simulink model "ThdynTest"  (R2013a)
settings: Solver=ode45  StartTime=0  StopTime=1  FixedStep=1e-3  RelTol=1e-5  AbsTol=1e-5
values from neighbouring files (symbols this model uses):
  B = [B1;B2]    [GensetRespOptimiztion.m]    (also in GensetRespOptimiztionTorstein.m; Init8RTFLEX68D.m = 0.68; init_MVM.m = 0.127)
  FExh0 = 0    [Init8RTFLEX68D.m]
  fs = 0.0683    [Init8RTFLEX68D.m]    (also in NOxProcessGUI.m = varargin{2}; initHybrid.m; initMV.m; init_MVM.m = 0.0682925799315)
  FScav0 = 0    [Init8RTFLEX68D.m]
  mCV = p*VCV / (R*T)    [ThdynCVTestScript.m]    (also in ThdynTest.m)
  mfCV = F*fs / (1+F*fs) * mCV    [ThdynCVTestScript.m]    (also in ThdynTest.m)
  pExh0 = pExhRef(caseInit)    [Init8RTFLEX68D.m]
  pScav0 = pScavRef(caseInit)    [Init8RTFLEX68D.m]
  RPM0 = simin(1,2)    [Init8RTFLEX68D.m]
  stroke = 2.72    [Init8RTFLEX68D.m]
  TExh0 = TExhRef(caseInit)    [Init8RTFLEX68D.m]
  TScav0 = TScavRef(caseInit)    [Init8RTFLEX68D.m]
  UCV = u*mCV    [ThdynCVTestScript.m]    (also in ThdynTest.m)
  VCV = 1.2    [ThdynCVTestScript.m]    (also in ThdynTest.m = 1)
undefined symbols (not defined in the file): alpha, beta, cAlpha, cAStartRef, cAVVDownRef, cAVVUpRef, cCylHT, dCALiftDown, dCALiftTopRef, dCALiftUp, Dp, DPhiMix, Ds, Dv, ECyl0, FCyl0, hn, lambdaCrank, liftDownRef, liftMax, liftUpRef, mbCyl0, mCp, mCyl0, mqfCycMax, nCyl, nPort, nStroke, pCyl0, phi0, phi0Mix, r, TCyl0, vCyl0, w, wiebePara, X, Y
libraries: EngineSysteSubmodel x12
settings Model: Creator=yum  LastModifiedBy=yum
settings DataIOCC: SaveFormat=StructureWithTime  ReturnWorkspaceOutputs=on

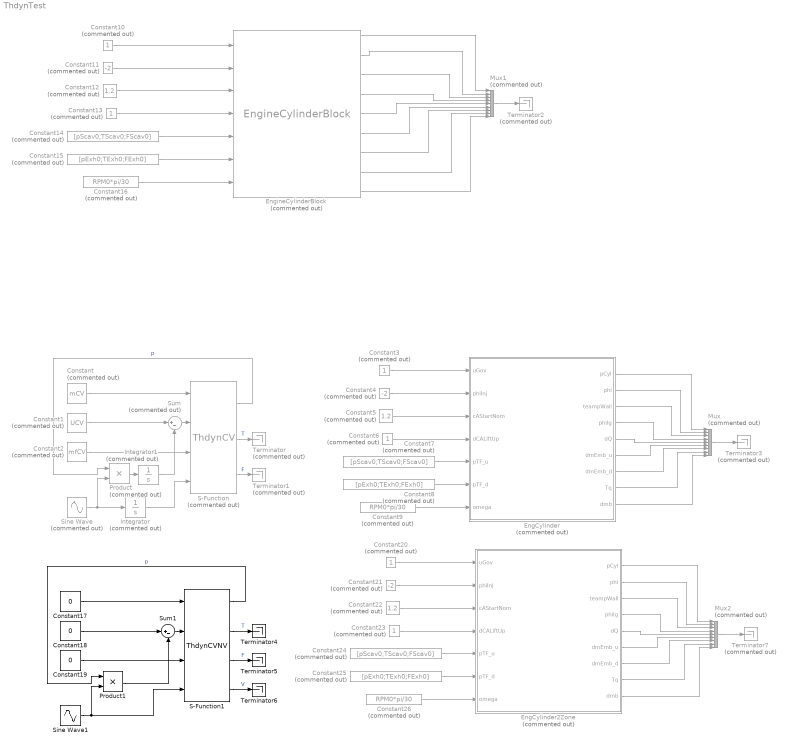
== system ThdynTest ==
  Constant : Constant  Commented=on  Value=mCV
  Constant1 : Constant  Commented=on  Value=UCV
  Constant{3,6,10,13,20,23} (6 alike) : Constant  Commented=on
  Constant11 : Constant  Commented=on  Value=-2
  Constant12 : Constant  Commented=on  Value=1.2
  Constant14 : Constant  Commented=on  Value=[pScav0;TScav0;FScav0]
  Constant15 : Constant  Commented=on  Value=[pExh0;TExh0;FExh0]
  Constant16 : Constant  Commented=on  Value=RPM0*pi/30
  Constant17 : Constant  Value=0
  Constant18 : Constant  Value=0
  Constant19 : Constant  Value=0
  Constant2 : Constant  Commented=on  Value=mfCV
  Constant21 : Constant  Commented=on  Value=-2
  Constant22 : Constant  Commented=on  Value=1.2
  Constant24 : Constant  Commented=on  Value=[pScav0;TScav0;FScav0]
  Constant25 : Constant  Commented=on  Value=[pExh0;TExh0;FExh0]
  Constant26 : Constant  Commented=on  Value=RPM0*pi/30
  Constant4 : Constant  Commented=on  Value=-2
  Constant5 : Constant  Commented=on  Value=1.2
  Constant7 : Constant  Commented=on  Value=[pScav0;TScav0;FScav0]
  Constant8 : Constant  Commented=on  Value=[pExh0;TExh0;FExh0]
  Constant9 : Constant  Commented=on  Value=RPM0*pi/30
  EngCylinder : Subsystem  Commented=on  AncestorBlock=EngineSysteSubmodel/EngCylinder  mask{fs=fs, nStroke=nStroke, hn=hn, nCyl=nCyl, iCyl=1, B=B, stroke=stroke, lambdaCrank=lambdaCrank, aCrank=stroke/2, X=X, Y=Y, r=r, nPort=nPort, liftMax=liftMax, Dv=Dv, beta=beta, w=w, Dp=Dp, Ds=Ds, cAVVUpRef=cAVVUpRef, cAVVDownRef=cAVVDownRef, liftUpRef=liftUpRef, liftDownRef=liftDownRef, cAStartRef=cAStartRef, dCALiftUp=dCALiftUp, dCALiftDown=dCALiftDown, dCALiftTopRef=dCALiftTopRef, mCp=mCp, cCylHT=cCylHT, cAlpha=cAlpha, mqfCycMax=mqfCycMax, wiebePara=wiebePara, phi0=phi0, m0=mCyl0, E0=ECyl0, mb0=mbCyl0, V0=vCyl0, phi0A=phi0, m0A=mCyl0, E0A=ECyl0, mb0A=mbCyl0, V0A=vCyl0}
      mask prompts: fs "Stoichiometric fuel-air ratio"; nStroke "Number of stroke"; hn "Lower heating value of the fuel [J/kg]"; nCyl "Number of cylinders"; iCyl "Cylinder number"; B "Bore of the cylinder [m]"; stroke "Stroke [m]"; lambdaCrank "Ratio of length of crank rod to connecting rod"; aCrank "Length of crank rod [m]"; X "Width of inport opening [m]"; Y "Height of inport opening [m]"; r "Raidus of fillet of the opening"; nPort "Number of ports [pcs]"; liftMax "Maximum valve lift [m]"; Dv "Valve head diameter [m]"; beta "Seat angle [rad]"; w "Valve seat width [m]"; Dp "Inner seat diameter [m]"; Ds "Stem diameter [m]"; cAVVUpRef "Crank angle array for opening [deg]"; cAVVDownRef "Crank angle array for closing [deg]"; liftUpRef "Normalized lift array for opening (0~1)"; liftDownRef "Normalized lift array for closing (0~1)"; cAStartRef "Nominal crank angle at start of valve lif [deg]"; dCALiftUp "Nominal duration of crank angle for valve opening [deg]"; dCALiftDown "Nominal duration of crank angle for valve closing [deg]"; dCALiftTopRef "Nominal duration of crank angle for valve open [deg]"; mCp "Heat capacity of the cylinder [J/K]"; cCylHT "Polynomial coefficient for heat rejection model from the cylinder (4 x 1)"; cAlpha "Fitting coefficient for convective heat transfer coefficient"; mqfCycMax "Maximum fuel mass injected per cycle [kg]"; wiebePara "3-Wiebe Parameters (9x1)"; phi0 "Initial crank angle [deg]"; m0 "Initial mass [kg]"; E0 "Initial internal energy [J]"; mb0 "Initial burned fuel mass [kg]"; V0 "Initial volume [m3]"; phi0A "Initial crank angle array [deg]"; m0A "Initial mass array [kg]"; E0A "Initial internal energy array [J]"; mb0A "Initial burned fuel mass array [kg]"; V0A "Initial volume array [m3]"
      mask init:
      | CylNo = uint8(iCyl);
      | if CylNo > 0 
      |     phi0 = phi0A(CylNo);
      |     m0 = m0A(CylNo);
      |     E0 = E0A(CylNo);
      |     mb0 = mb0A(CylNo);
      |     V0 = V0A(CylNo);
      | else
      |     phi0 = phi0A(1);
      |     m0 = m0A(1);
      |     E0 = E0A(1);
      |     mb0 = mb0A(1);
      |     V0 = V0A(1);
      | end;
      mask TypeOptions fs: ThdynCV_VarVol1/fs | IntakePort1/fs | ExhValve/fs
      mask TypeOptions nStroke: IntakePort1/nStroke
      mask TypeOptions hn: ROHR1/hn
      mask TypeOptions nCyl: EngCylHeatTransfer/nCyl
      mask TypeOptions B: CrankMechKinematic/B | EngCylHeatTransfer/B
      mask TypeOptions stroke: CrankMechKinematic/stroke | EngCylHeatTransfer/stroke | IntakePort1/stroke
      mask TypeOptions lambdaCrank: IntakePort1/lambdaCrank | CrankMechKinematic/lambdaCrank
      mask TypeOptions aCrank: IntakePort1/aCrank
      mask TypeOptions X: IntakePort1/X
      mask TypeOptions Y: IntakePort1/Y
      mask TypeOptions r: IntakePort1/r
      mask TypeOptions nPort: IntakePort1/nPort
      mask TypeOptions liftMax: ExhValve/liftMax
      mask TypeOptions Dv: ExhValve/Dv
      mask TypeOptions beta: ExhValve/beta
      mask TypeOptions w: ExhValve/w
      mask TypeOptions Dp: ExhValve/Dp
      mask TypeOptions Ds: ExhValve/Ds
      mask TypeOptions cAVVUpRef: ExhValve/cAVVUpRef
      mask TypeOptions cAVVDownRef: ExhValve/cAVVDownRef
      mask TypeOptions liftUpRef: ExhValve/liftUpRef
      mask TypeOptions liftDownRef: ExhValve/liftDownRef
      mask TypeOptions cAStartRef: ExhValve/cAStartRef
      mask TypeOptions dCALiftUp: ExhValve/dCALiftUp
      mask TypeOptions dCALiftDown: ExhValve/dCALiftDown
      mask TypeOptions dCALiftTopRef: ExhValve/dCALiftTopRef
      mask TypeOptions mCp: EngCylHeatTransfer/mCp
      mask TypeOptions cCylHT: EngCylHeatTransfer/cCylHT
      mask TypeOptions cAlpha: EngCylHeatTransfer/cAlpha
      mask TypeOptions mqfCycMax: ROHR1/mqfCycMax
      mask TypeOptions wiebePara: ROHR1/wiebePara
      mask TypeOptions phi0: CrankMechKinematic/phi0
      mask TypeOptions m0: ThdynCV_VarVol1/m0
      mask TypeOptions E0: ThdynCV_VarVol1/E0
      mask TypeOptions mb0: ThdynCV_VarVol1/mb0
      mask TypeOptions V0: ThdynCV_VarVol1/V0
  EngCylinder2Zone : Subsystem  Commented=on  mask{fs=fs, nStroke=nStroke, hn=hn, nCyl=nCyl, iCyl=1, B=B, stroke=stroke, lambdaCrank=lambdaCrank, aCrank=stroke/2, X=X, Y=Y, r=r, nPort=nPort, liftMax=liftMax, Dv=Dv, beta=beta, w=w, Dp=Dp, Ds=Ds, cAVVUpRef=cAVVUpRef, cAVVDownRef=cAVVDownRef, liftUpRef=liftUpRef, liftDownRef=liftDownRef, cAStartRef=cAStartRef, dCALiftUp=dCALiftUp, dCALiftDown=dCALiftDown, dCALiftTopRef=dCALiftTopRef, mCp=mCp, cCylHT=cCylHT, cAlpha=cAlpha, mqfCycMax=mqfCycMax, wiebePara=wiebePara, DPhiMix=DPhiMix, phiMix0=phi0Mix, alpha=alpha, phi0=phi0, p0=mCyl0, T0=ECyl0, F0=mbCyl0, V0=vCyl0, phi0A=phi0, p0A=pCyl0, T0A=TCyl0, F0A=FCyl0, V0A=vCyl0}
      mask prompts: fs "Stoichiometric fuel-air ratio"; nStroke "Number of stroke"; hn "Lower heating value of the fuel [J/kg]"; nCyl "Number of cylinders"; iCyl "Cylinder number"; B "Bore of the cylinder [m]"; stroke "Stroke [m]"; lambdaCrank "Ratio of length of crank rod to connecting rod"; aCrank "Length of crank rod [m]"; X "Width of inport opening [m]"; Y "Height of inport opening [m]"; r "Raidus of fillet of the opening"; nPort "Number of ports [pcs]"; liftMax "Maximum valve lift [m]"; Dv "Valve head diameter [m]"; beta "Seat angle [rad]"; w "Valve seat width [m]"; Dp "Inner seat diameter [m]"; Ds "Stem diameter [m]"; cAVVUpRef "Crank angle array for opening [deg]"; cAVVDownRef "Crank angle array for closing [deg]"; liftUpRef "Normalized lift array for opening (0~1)"; liftDownRef "Normalized lift array for closing (0~1)"; cAStartRef "Nominal crank angle at start of valve lif [deg]"; dCALiftUp "Nominal duration of crank angle for valve opening [deg]"; dCALiftDown "Nominal duration of crank angle for valve closing [deg]"; dCALiftTopRef "Nominal duration of crank angle for valve open [deg]"; mCp "Heat capacity of the cylinder [J/K]"; cCylHT "Polynomial coefficient for heat rejection model from the cylinder (4 x 1)"; cAlpha "Fitting coefficient for convective heat transfer coefficient"; mqfCycMax "Maximum fuel mass injected per cycle [kg]"; wiebePara "3-Wiebe Parameters (9x1)"; DPhiMix "Duration of mixing from burned zone to unburned zone [deg]"; phiMix0 "Start of mixing from burned zone to unburend [deg]"; alpha "Ratio of burned mass to unburned during gas exchange"; phi0 "Initial crank angle [deg]"; p0 "Initial pressure [Pa]"; T0 "Initial temperature [K]"; F0 "Initial fuel-air equivalent ratio"; V0 "Initial volume [m3]"; phi0A "Initial crank angle array [deg]"; p0A "Initial pressure array [Pa]"; T0A "Initial temperature array [K]"; F0A "Initial fuel-air equivalent ratio array"; V0A "Initial volume array [m3]"
      mask init:
      | CylNo = uint8(iCyl);
      | if CylNo > 0 
      |     phi0 = phi0A(CylNo);
      |     p0 = p0A(CylNo);
      |     T0 = T0A(CylNo);
      |     F0 = F0A(CylNo);
      |     V0 = V0A(CylNo);
      | else
      |     phi0 = phi0A(1);
      |     p0 = p0A(1);
      |     T0 = T0A(1);
      |     F0 = F0A(1);
      |     V0 = V0A(1);
      | end;
      mask TypeOptions fs: IntakePort1/fs | ExhValve/fs | ThdynCV2ZoneBG/fs
      mask TypeOptions nStroke: IntakePort1/nStroke
      mask TypeOptions hn: ROHR1/hn | ThdynCV2ZoneBG/hn
      mask TypeOptions nCyl: EngCylHeatTransfer/nCyl
      mask TypeOptions B: CrankMechKinematic/B | EngCylHeatTransfer/B
      mask TypeOptions stroke: CrankMechKinematic/stroke | EngCylHeatTransfer/stroke | IntakePort1/stroke
      mask TypeOptions lambdaCrank: IntakePort1/lambdaCrank | CrankMechKinematic/lambdaCrank
      mask TypeOptions aCrank: IntakePort1/aCrank
      mask TypeOptions X: IntakePort1/X
      mask TypeOptions Y: IntakePort1/Y
      mask TypeOptions r: IntakePort1/r
      mask TypeOptions nPort: IntakePort1/nPort
      mask TypeOptions liftMax: ExhValve/liftMax
      mask TypeOptions Dv: ExhValve/Dv
      mask TypeOptions beta: ExhValve/beta
      mask TypeOptions w: ExhValve/w
      mask TypeOptions Dp: ExhValve/Dp
      mask TypeOptions Ds: ExhValve/Ds
      mask TypeOptions cAVVUpRef: ExhValve/cAVVUpRef
      mask TypeOptions cAVVDownRef: ExhValve/cAVVDownRef
      mask TypeOptions liftUpRef: ExhValve/liftUpRef
      mask TypeOptions liftDownRef: ExhValve/liftDownRef
      mask TypeOptions cAStartRef: ExhValve/cAStartRef
      mask TypeOptions dCALiftUp: ExhValve/dCALiftUp
      mask TypeOptions dCALiftDown: ExhValve/dCALiftDown
      mask TypeOptions dCALiftTopRef: ExhValve/dCALiftTopRef
      mask TypeOptions mCp: EngCylHeatTransfer/mCp
      mask TypeOptions cCylHT: EngCylHeatTransfer/cCylHT
      mask TypeOptions cAlpha: EngCylHeatTransfer/cAlpha
      mask TypeOptions mqfCycMax: ROHR1/mqfCycMax
      mask TypeOptions wiebePara: ROHR1/wiebePara
      mask TypeOptions DPhiMix: ThdynCV2ZoneBG/DPhiMix
      mask TypeOptions phiMix0: ThdynCV2ZoneBG/phiMix0
      mask TypeOptions alpha: ThdynCV2ZoneBG/alpha
      mask TypeOptions phi0: CrankMechKinematic/phi0
      mask TypeOptions p0: ThdynCV2ZoneBG/p0
      mask TypeOptions T0: ThdynCV2ZoneBG/T0
      mask TypeOptions F0: ThdynCV2ZoneBG/F0
      mask TypeOptions V0: ThdynCV2ZoneBG/V0
  EngineCylinderBlock : EngineSysteSubmodel/EngineCylinderBlock  Commented=on  fs=fs  nStroke=nStroke  hn=hn  nCyl=nCyl  B=B  stroke=stroke  lambdaCrank=lambdaCrank  aCrank=stroke/2  X=X  Y=Y  r=r  nPort=nPort  liftMax=liftMax  Dv=Dv  beta=beta  w=w  Dp=Dp  Ds=Ds  cAVVUpRef=cAVVUpRef  cAVVDownRef=cAVVDownRef  liftUpRef=liftUpRef  liftDownRef=liftDownRef  cAStartRef=cAStartRef  dCALiftUp=dCALiftUp  dCALiftDown=dCALiftDown  dCALiftTopRef=dCALiftTopRef  mCp=mCp  cCylHT=cCylHT  cAlpha=cAlpha  mqfCycMax=mqfCycMax  wiebePara=wiebePara  phi0A=phi0rad  m0A=mCyl0  E0A=ECyl0  mb0A=mbCyl0  V0A=vCyl0
  Integrator : Integrator  Commented=on  InitialCondition=VCV
  Integrator1 : Integrator  Commented=on
  Mux : Mux  Commented=on  Inputs=9
  Mux1 : Mux  Commented=on  Inputs=9
  Mux2 : Mux  Commented=on  Inputs=9
  Product : Product  Commented=on
  Product1 : Product
  S-Function : S-Function  Commented=on  FunctionName=ThdynCV  Parameters=fs  EnableBusSupport=off
  S-Function1 : S-Function  FunctionName=ThdynCVNV  Parameters=fs,mCV,UCV,mfCV,VCV  EnableBusSupport=off
  Sine Wave : Sin  Commented=on  Amplitude=-0.25*10  Frequency=10  SampleTime=0
  Sine Wave1 : Sin  Amplitude=-0.25*10  Frequency=10  SampleTime=0
  Sum : Sum  Commented=on  Inputs=|+-
  Sum1 : Sum  Inputs=|+-
  Terminator{,1..3,7} (5 alike) : Terminator  Commented=on
  Terminator4 : Terminator
  Terminator5 : Terminator
  Terminator6 : Terminator
  wires:
  Constant/1 -> S-Function/1
  Constant1/1 -> Sum/1
  Constant2/1 -> S-Function/3
  S-Function/1 -> Product/1  "p"
  Sine Wave/1 -> Product/2, Integrator/1
  Integrator/1 -> S-Function/4
  Sum/1 -> S-Function/2
  Product/1 -> Integrator1/1
  Integrator1/1 -> Sum/2
  S-Function/2 -> Terminator/1  "T"
  S-Function/3 -> Terminator1/1  "F"
  Constant3/1 -> EngCylinder/1(uGov)
  Constant4/1 -> EngCylinder/2(phiInj)
  Constant5/1 -> EngCylinder/3(cAStartNom)
  Constant6/1 -> EngCylinder/4(dCALiftUp)
  Constant7/1 -> EngCylinder/5(pTF_u)
  Constant8/1 -> EngCylinder/6(pTF_d)
  Constant9/1 -> EngCylinder/7(omega)
  EngCylinder/1(pCyl) -> Mux/1
  EngCylinder/2(phi) -> Mux/2
  EngCylinder/3(teampWall) -> Mux/3
  EngCylinder/4(phiIg) -> Mux/4
  EngCylinder/5(dQ) -> Mux/5
  EngCylinder/6(dmEmb_u) -> Mux/6
  EngCylinder/7(dmEmb_d) -> Mux/7
  EngCylinder/8(Tq) -> Mux/8
  EngCylinder/9(dmb) -> Mux/9
  Mux/1 -> Terminator3/1
  Constant10/1 -> EngineCylinderBlock/1
  Constant11/1 -> EngineCylinderBlock/2
  Constant12/1 -> EngineCylinderBlock/3
  Constant13/1 -> EngineCylinderBlock/4
  Constant14/1 -> EngineCylinderBlock/5
  Constant15/1 -> EngineCylinderBlock/6
  Constant16/1 -> EngineCylinderBlock/7
  EngineCylinderBlock/1 -> Mux1/1
  EngineCylinderBlock/2 -> Mux1/2
  EngineCylinderBlock/3 -> Mux1/3
  EngineCylinderBlock/4 -> Mux1/4
  EngineCylinderBlock/5 -> Mux1/5
  EngineCylinderBlock/6 -> Mux1/6
  EngineCylinderBlock/7 -> Mux1/7
  EngineCylinderBlock/8 -> Mux1/8
  EngineCylinderBlock/9 -> Mux1/9
  Mux1/1 -> Terminator2/1
  Constant17/1 -> S-Function1/1
  Constant18/1 -> Sum1/1
  Constant19/1 -> S-Function1/3
  S-Function1/1 -> Product1/1  "p"
  Sine Wave1/1 -> S-Function1/4, Product1/2
  Sum1/1 -> S-Function1/2
  Product1/1 -> Sum1/2
  S-Function1/2 -> Terminator4/1  "T"
  S-Function1/3 -> Terminator5/1  "F"
  S-Function1/4 -> Terminator6/1  "V"
  Constant20/1 -> EngCylinder2Zone/1(uGov)
  Constant21/1 -> EngCylinder2Zone/2(phiInj)
  Constant22/1 -> EngCylinder2Zone/3(cAStartNom)
  Constant23/1 -> EngCylinder2Zone/4(dCALiftUp)
  Constant24/1 -> EngCylinder2Zone/5(pTF_u)
  Constant25/1 -> EngCylinder2Zone/6(pTF_d)
  Constant26/1 -> EngCylinder2Zone/7(omega)
  EngCylinder2Zone/1(pCyl) -> Mux2/1
  EngCylinder2Zone/2(phi) -> Mux2/2
  EngCylinder2Zone/3(teampWall) -> Mux2/3
  EngCylinder2Zone/4(phiIg) -> Mux2/4
  EngCylinder2Zone/5(dQ) -> Mux2/5
  EngCylinder2Zone/6(dmEmb_u) -> Mux2/6
  EngCylinder2Zone/7(dmEmb_d) -> Mux2/7
  EngCylinder2Zone/8(Tq) -> Mux2/8
  EngCylinder2Zone/9(dmb) -> Mux2/9
  Mux2/1 -> Terminator7/1

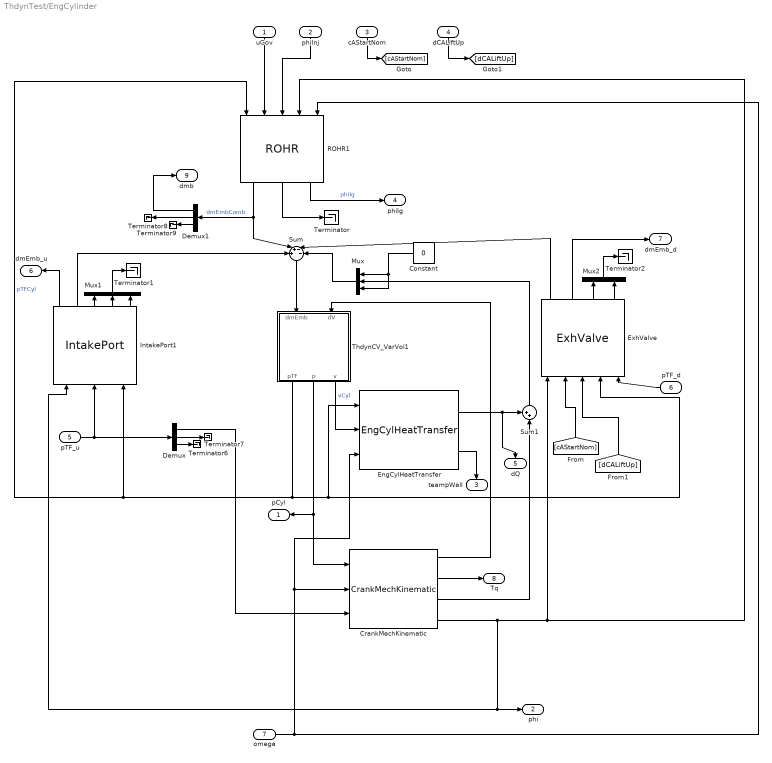
== system ThdynTest/EngCylinder ==
  uGov : Inport
  phiInj : Inport  Port=2
  cAStartNom : Inport  Port=3
  dCALiftUp : Inport  Port=4
  pTF_u : Inport  Port=5
  pTF_d : Inport  Port=6
  omega : Inport  Port=7
  Constant : Constant  Value=0
  CrankMechKinematic : EngineSysteSubmodel/CrankMechKinematic  phi0=phi0  B=B  stroke=stroke  lambdaCrank=lambdaCrank
  Demux : Demux  Outputs=3
  Demux1 : Demux  Outputs=3
  EngCylHeatTransfer : EngineSysteSubmodel/EngCylHeatTransfer  stroke=stroke  B=B  cAlpha=cAlpha  mCp=mCp  cCylHT=cCylHT  nCyl=nCyl  tempWall0=600
  ExhValve : EngineSysteSubmodel/ExhValve  fs=fs  cAVVUpRef=cAVVUpRef  cAVVDownRef=cAVVDownRef  liftUpRef=liftUpRef  liftDownRef=liftDownRef  cAStartRef=cAStartRef  dCALiftUp=dCALiftUp  dCALiftDown=dCALiftDown  dCALiftTopRef=dCALiftTopRef  liftMax=liftMax  Dv=Dv  beta=beta  w=w  Dp=Dp  Ds=Ds
  IntakePort1 : EngineSysteSubmodel/IntakePort  fs=fs  nStroke=nStroke  aCrank=aCrank  lambdaCrank=lambdaCrank  X=X  Y=Y  r=r  nPort=nPort  stroke=stroke
  Mux : Mux  Inputs=3
  Mux1 : Mux  Inputs=3
  Mux2 : Mux  Inputs=2
  ROHR1 : EngineSysteSubmodel/ROHR  mqfCycMax=mqfCycMax  wiebePara=wiebePara  hn=hn
  Sum : Sum  Inputs=++--
  Sum1 : Sum  Inputs=++|
  Terminator{,1..2,6..9} (7 alike) : Terminator
  ThdynCV_VarVol1 : Subsystem  AncestorBlock=EngineSysteSubmodel/ThdynCV_VarVol  mask{fs=fs, m0=m0, E0=E0, mb0=mb0, V0=V0}
      mask prompts: fs "Stoichiometric fuel-air ratio"; m0 "Initial mass (kg)"; E0 "Initial internal energy (J)"; mb0 "Initial burned fuel mass (kg)"; V0 "Initial volume (m3)"
  pCyl : Outport
  phi : Outport  Port=2
  teampWall : Outport  Port=3
  phiIg : Outport  Port=4
  dQ : Outport  Port=5
  dmEmb_u : Outport  Port=6
  dmEmb_d : Outport  Port=7
  Tq : Outport  Port=8
  dmb : Outport  Port=9
  wires:
  Demux1/3 -> Terminator9/1
  Demux1/2 -> Terminator8/1
  Demux1/1 -> dmb/1
  ROHR1/1 -> Demux1/1, Sum/2  "dmEmbComb"
  IntakePort1/2 -> Sum/1
  ExhValve/1 -> Sum/3
  Sum/1 -> ThdynCV_VarVol1/1(dmEmb)
  ThdynCV_VarVol1/1(pTF) -> EngCylHeatTransfer/1, ExhValve/4, ROHR1/1, IntakePort1/3  "pTFCyl"
  ThdynCV_VarVol1/2(p) -> pCyl/1, CrankMechKinematic/1
  CrankMechKinematic/4 -> ROHR1/4, ExhValve/1, phi/1, IntakePort1/1
  CrankMechKinematic/1 -> ThdynCV_VarVol1/2(dV)
  uGov/1 -> ROHR1/2
  CrankMechKinematic/3 -> Sum1/2
  Demux/1 -> CrankMechKinematic/3
  CrankMechKinematic/2 -> Tq/1
  phiInj/1 -> ROHR1/3
  pTF_d/1 -> ExhValve/5
  omega/1 -> EngCylHeatTransfer/3, CrankMechKinematic/2, ROHR1/5
  ROHR1/2 -> Terminator/1
  IntakePort1/1 -> dmEmb_u/1
  pTF_u/1 -> IntakePort1/2, Demux/1
  ThdynCV_VarVol1/3(v) -> EngCylHeatTransfer/2  "vCyl"
  EngCylHeatTransfer/1 -> Sum1/1, dQ/1
  Sum1/1 -> Mux/2
  Mux/1 -> Sum/4
  Constant/1 -> Mux/3, Mux/1
  Demux/2 -> Terminator6/1
  Demux/3 -> Terminator7/1
  EngCylHeatTransfer/2 -> teampWall/1
  ROHR1/3 -> phiIg/1  "phiIg"
  IntakePort1/3 -> Mux1/1
  IntakePort1/4 -> Mux1/2
  IntakePort1/5 -> Mux1/3
  Mux1/1 -> Terminator1/1
  ExhValve/3 -> Mux2/1
  ExhValve/4 -> Mux2/2
  Mux2/1 -> Terminator2/1
  ExhValve/2 -> dmEmb_d/1
  cAStartNom/1 -> [cAStartNom]
  dCALiftUp/1 -> [dCALiftUp]
  [cAStartNom] -> ExhValve/2
  [dCALiftUp] -> ExhValve/3

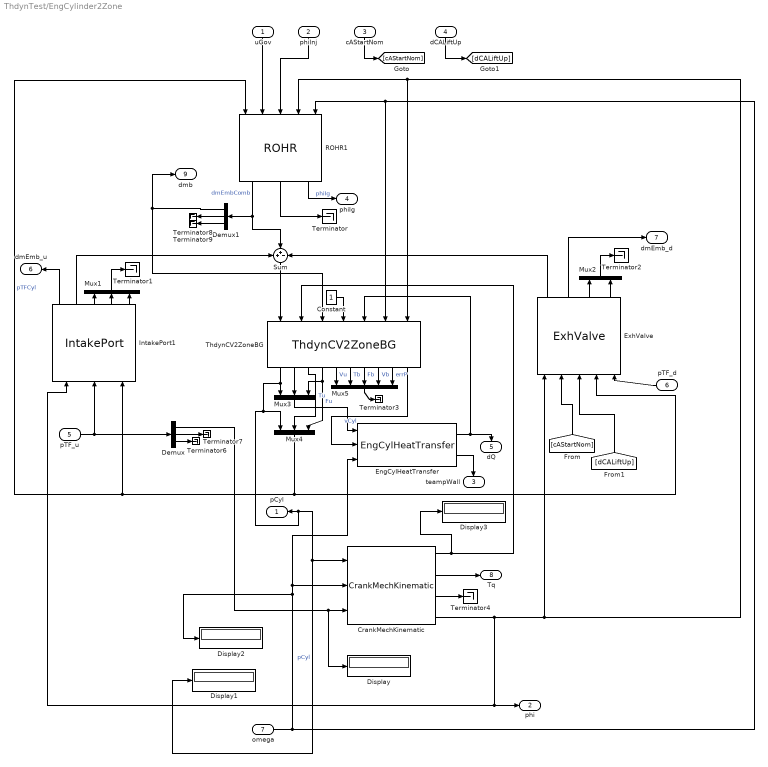
== system ThdynTest/EngCylinder2Zone ==
  uGov : Inport
  phiInj : Inport  Port=2
  cAStartNom : Inport  Port=3
  dCALiftUp : Inport  Port=4
  pTF_u : Inport  Port=5
  pTF_d : Inport  Port=6
  omega : Inport  Port=7
  Constant : Constant
  CrankMechKinematic : EngineSysteSubmodel/CrankMechKinematic  phi0=phi0  B=B  stroke=stroke  lambdaCrank=lambdaCrank
  Demux : Demux  Outputs=3
  Demux1 : Demux  Outputs=3
  Display{,1..3} (4 alike) : Display
  EngCylHeatTransfer : EngineSysteSubmodel/EngCylHeatTransfer  stroke=stroke  B=B  cAlpha=cAlpha  mCp=mCp  cCylHT=cCylHT  nCyl=nCyl  tempWall0=600
  ExhValve : EngineSysteSubmodel/ExhValve  fs=fs  cAVVUpRef=cAVVUpRef  cAVVDownRef=cAVVDownRef  liftUpRef=liftUpRef  liftDownRef=liftDownRef  cAStartRef=cAStartRef  dCALiftUp=dCALiftUp  dCALiftDown=dCALiftDown  dCALiftTopRef=dCALiftTopRef  liftMax=liftMax  Dv=Dv  beta=beta  w=w  Dp=Dp  Ds=Ds
  IntakePort1 : EngineSysteSubmodel/IntakePort  fs=fs  nStroke=nStroke  aCrank=aCrank  lambdaCrank=lambdaCrank  X=X  Y=Y  r=r  nPort=nPort  stroke=stroke
  Mux1 : Mux  Inputs=3
  Mux2 : Mux  Inputs=2
  Mux3 : Mux  Inputs=3
  Mux4 : Mux  Inputs=3
  Mux5 : Mux  Inputs=5
  ROHR1 : EngineSysteSubmodel/ROHR  mqfCycMax=mqfCycMax  wiebePara=wiebePara  hn=hn
  Sum : Sum  Inputs=++-
  Terminator{,1..4,6..9} (9 alike) : Terminator
  ThdynCV2ZoneBG : EngineSysteSubmodel/ThdynCV2ZoneBG  fs=fs  DPhiMix=DPhiMix  phiMix0=phiMix0  alpha=alpha  hn=hn  p0=p0  T0=T0  F0=F0  V0=V0
  pCyl : Outport
  phi : Outport  Port=2
  teampWall : Outport  Port=3
  phiIg : Outport  Port=4
  dQ : Outport  Port=5
  dmEmb_u : Outport  Port=6
  dmEmb_d : Outport  Port=7
  Tq : Outport  Port=8
  dmb : Outport  Port=9
  wires:
  Demux1/3 -> Terminator9/1
  Demux1/2 -> Terminator8/1
  Demux1/1 -> ThdynCV2ZoneBG/3, dmb/1
  ROHR1/1 -> Sum/2, Demux1/1  "dmEmbComb"
  IntakePort1/2 -> Sum/1
  ExhValve/1 -> Sum/3
  Sum/1 -> ThdynCV2ZoneBG/1
  Mux4/1 -> ROHR1/1, IntakePort1/3, ExhValve/4  "pTFCyl"
  ThdynCV2ZoneBG/1 -> Mux4/1, Display1/1, CrankMechKinematic/1, pCyl/1, Mux3/1  "pCyl"
  CrankMechKinematic/4 -> ROHR1/4, ThdynCV2ZoneBG/7, ExhValve/1, phi/1, IntakePort1/1
  CrankMechKinematic/1 -> Display3/1, ThdynCV2ZoneBG/2
  uGov/1 -> ROHR1/2
  Demux/1 -> Display/1, CrankMechKinematic/3
  CrankMechKinematic/2 -> Tq/1
  phiInj/1 -> ROHR1/3
  pTF_d/1 -> ExhValve/5
  omega/1 -> EngCylHeatTransfer/3, CrankMechKinematic/2, Display2/1, ThdynCV2ZoneBG/6, ROHR1/5
  ROHR1/2 -> Terminator/1
  IntakePort1/1 -> dmEmb_u/1
  pTF_u/1 -> IntakePort1/2, Demux/1
  ThdynCV2ZoneBG/10 -> EngCylHeatTransfer/2  "vCyl"
  EngCylHeatTransfer/1 -> dQ/1, ThdynCV2ZoneBG/5
  Demux/2 -> Terminator6/1
  Demux/3 -> Terminator7/1
  EngCylHeatTransfer/2 -> teampWall/1
  ROHR1/3 -> phiIg/1  "phiIg"
  IntakePort1/3 -> Mux1/1
  IntakePort1/4 -> Mux1/2
  IntakePort1/5 -> Mux1/3
  Mux1/1 -> Terminator1/1
  ExhValve/3 -> Mux2/1
  ExhValve/4 -> Mux2/2
  Mux2/1 -> Terminator2/1
  ExhValve/2 -> dmEmb_d/1
  cAStartNom/1 -> [cAStartNom]
  dCALiftUp/1 -> [dCALiftUp]
  [cAStartNom] -> ExhValve/2
  [dCALiftUp] -> ExhValve/3
  ThdynCV2ZoneBG/2 -> Mux3/2
  ThdynCV2ZoneBG/4 -> Mux4/3, Mux3/3  "Fu"
  Mux3/1 -> EngCylHeatTransfer/1
  ThdynCV2ZoneBG/3 -> Mux4/2  "Tu"
  ThdynCV2ZoneBG/6 -> Mux5/2  "Tb"
  ThdynCV2ZoneBG/5 -> Mux5/1  "Vu"
  ThdynCV2ZoneBG/7 -> Mux5/3  "Fb"
  ThdynCV2ZoneBG/8 -> Mux5/4  "Vb"
  ThdynCV2ZoneBG/9 -> Mux5/5  "errP"
  Mux5/1 -> Terminator3/1
  CrankMechKinematic/3 -> Terminator4/1
  Constant/1 -> ThdynCV2ZoneBG/4

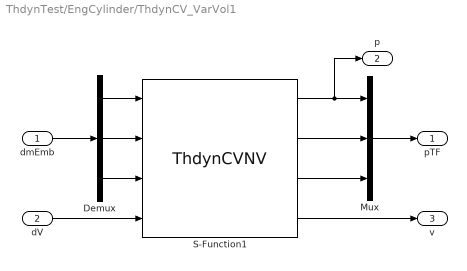
== system ThdynTest/EngCylinder/ThdynCV_VarVol1 ==
  dmEmb : Inport
  dV : Inport  Port=2
  Demux : Demux  Outputs=3
  Mux : Mux  Inputs=3
  S-Function1 : S-Function  FunctionName=ThdynCVNV  Parameters=fs,m0,E0,mb0,V0  EnableBusSupport=off
  pTF : Outport
  p : Outport  Port=2
  v : Outport  Port=3
  wires:
  Demux/1 -> S-Function1/1
  dmEmb/1 -> Demux/1
  Demux/2 -> S-Function1/2
  Demux/3 -> S-Function1/3
  dV/1 -> S-Function1/4
  S-Function1/1 -> p/1, Mux/1
  S-Function1/2 -> Mux/2
  S-Function1/3 -> Mux/3
  S-Function1/4 -> v/1
  Mux/1 -> pTF/1
